simulink model "Cart_Pole_Simulink"  (R2021b)
settings: Solver=VariableStepAuto  StartTime=0.0  StopTime=10.0  RelTol=1e-3
values from neighbouring files (symbols this model uses):
  A = [0                   1                   0  0 ... (first row only)    [state_space_cartpole_simulink.m]
  B = [0; (I+m*l^2)/denom; 0; m*l/denom]    [state_space_cartpole_simulink.m]
  K = place(A,B,lambda)    [state_space_cartpole_simulink.m]
settings Model: Creator=mithu  LastModifiedBy=mithu

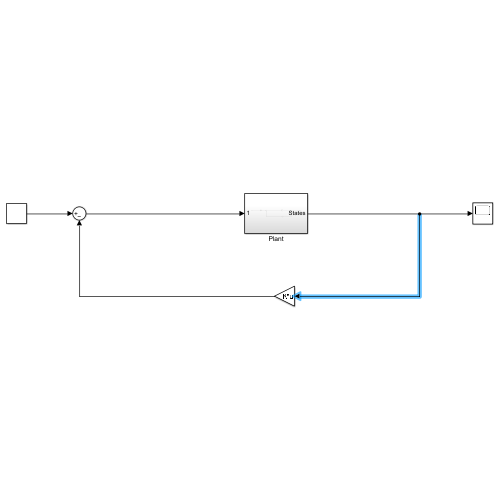
[thumbnail: Simulink's stored preview of the top-level diagram]
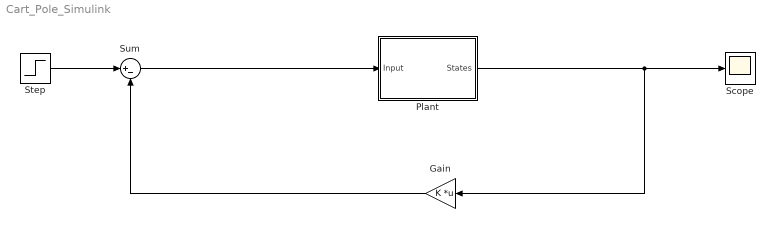
== system Cart_Pole_Simulink ==
  Gain : Gain  Gain=K  Multiplication=Matrix(K*u)
  Plant : Subsystem
  Scope : Scope
  Step : Step  SampleTime=0
  Sum : Sum  Inputs=|+-
  wires:
  Plant/1(States) -> Gain/1, Scope/1
  Step/1 -> Sum/1
  Sum/1 -> Plant/1(Input)
  Gain/1 -> Sum/2

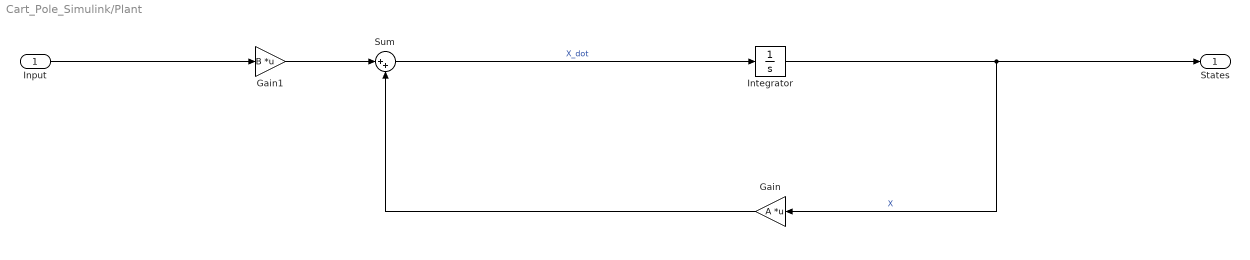
== system Cart_Pole_Simulink/Plant ==
  Input : Inport
  Gain : Gain  Gain=A  Multiplication=Matrix(K*u)
  Gain1 : Gain  Gain=B  Multiplication=Matrix(K*u)
  Integrator : Integrator
  Sum : Sum  Inputs=|++
  States : Outport
  wires:
  Sum/1 -> Integrator/1  "X_dot"
  Gain1/1 -> Sum/1
  Integrator/1 -> States/1, Gain/1  "X"
  Input/1 -> Gain1/1
  Gain/1 -> Sum/2
